simulink model "RAM_address_definition"  (R2020a)
settings: Solver=FixedStepDiscrete  StartTime=0.0  StopTime=840000  RelTol=1e-3
libraries: simulink x12, hdlsllib x8
settings Model: FPTRunName=FPA_Reference  PacingRate=40  Creator=BuccelliLab  LastModifiedBy=diflo
settings SolverCC: AutoInsertRateTranBlk=on  MinimalZcImpactIntegration=on
settings DataIOCC: LimitDataPoints=on  SaveOutput=off  SaveTime=off  ReturnWorkspaceOutputs=off
settings OptimizationCC: BlockReduction=off  ConditionallyExecuteInputs=off  DefaultParameterBehavior=Inlined  LifeSpan=inf
settings DebuggingCC: SignalRangeChecking=warning  ReadBeforeWriteMsg=DisableAll  WriteAfterWriteMsg=DisableAll  WriteAfterReadMsg=DisableAll  AlgebraicLoopMsg=error  MultiTaskDSMMsg=none  SingleTaskRateTransMsg=error  ParameterDowncastMsg=warning  ParameterOverflowMsg=warning  AllowSymbolicDim=off  StrictBusMsg=ErrorOnBusTreatedAsVector  SFUnexpectedBacktrackingDiag=warning  SFNoUnconditionalDefaultTransitionDiag=warning  SFExecutionAtInitializationDiag=none  ArithmeticOperatorsInVariantConditions=warning
settings HardwareCC: ProdBitPerPointer=32  ProdBitPerSizeT=32  ProdBitPerPtrDiffT=32  ProdLargestAtomicFloat=None  ProdIntDivRoundTo=Undefined  ProdEndianess=Unspecified  ProdWordSize=32  ProdHWDeviceType=ASIC/FPGA->ASIC/FPGA  TargetBitPerPointer=64  TargetBitPerSizeT=64  TargetBitPerPtrDiffT=64  TargetLongLongMode=on  TargetIntDivRoundTo=Zero  TargetEndianess=LittleEndian  TargetWordSize=64  TargetHWDeviceType=Custom Processor->MATLAB Host Computer  ProdEqTarget=off
settings ModelReferenceCC: UpdateModelReferenceTargets=IfOutOfDate
settings SFSimCC: SFSimEcho=off  SimUseLocalCustomCode=off  CustomCodeUndefinedFunction=UseInterfaceOnly
settings RTWCC: RTWUseLocalCustomCode=off
settings CodeAppCC: StateflowObjectComments=on
settings GRTTargetCC: TargetLangStandard=C89/C90 (ANSI)
settings ConfigComp: CovScope=ReferencedModels  CovMetricSettings=dw  CovHtmlReporting=on  CovSaveCumulativeToWorkspaceVar=on  CovSaveSingleToWorkspaceVar=on  CovExternalEMLEnable=off  CovSFcnEnable=off

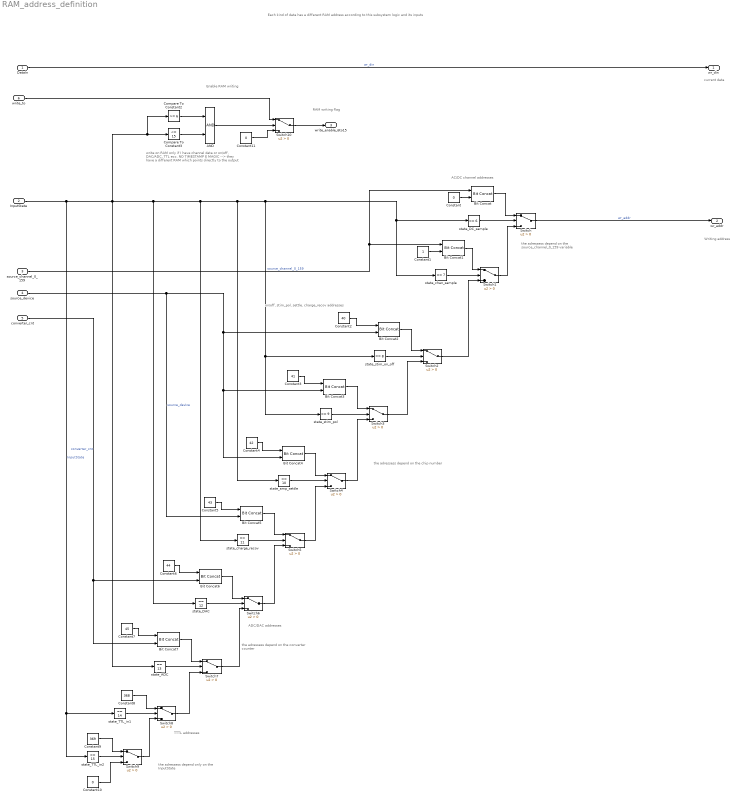
== system RAM_address_definition ==
  note: the adressess depend on the chip number
  note: Each kind of data has a different RAM
      | address according to this subsystem logic
      | and its inputs
  note: AC/DC channel addresses
  note: Writing address
  note: current data
  note: RAM writing flag
  note: write on RAM only if I have channel data or on/off,
      | DAC/ADC, TTL ecc.
      | NO TIMESTAMP E MAGIC --> they have a different
      | RAM which points directly to the output
  note: on/off, stim_pol, settle, charge_recov addresses
  note: ADC/DAC addresses
  note: TTTL addresses
  note: the adressess depend on the converter
      | counter
  note: the adressess depend only on the
      | InputState
  note: the adressess depend on the
      | source_channel_0_159 variable
  note: Enable RAM writing
  DataIn : Inport  OutDataTypeStr=uint16  PortDimensions=1  SampleTime=[1,0]
  InputState : Inport  Port=2  OutDataTypeStr=uint8  PortDimensions=1  SampleTime=[1,0]
  source_channel_0_159 : Inport  Port=3  OutDataTypeStr=uint8  PortDimensions=1  SampleTime=[1,0]
  source_device : Inport  Port=4  OutDataTypeStr=fixdt(0,3,0)  PortDimensions=1  SampleTime=[1,0]
  converter_cnt : Inport  Port=5  OutDataTypeStr=fixdt(0,3,0)  PortDimensions=1  SampleTime=[1,0]
  write_to : Inport  Port=6  OutDataTypeStr=boolean  PortDimensions=1  SampleTime=[1,0]
  AND : Logic  IconShape=distinctive  AllPortsSameDT=off  OutDataTypeStr=boolean
  Bit Concat{,1..7} (8 alike) : hdlsllib/Logic and Bit Operations/Bit Concat  numInputs=2
  Compare To Constant2 : simulink/Logic and Bit Operations/Compare To Constant  relop=>=  const=6  OutDataTypeStr=boolean
  Compare To Constant3 : simulink/Logic and Bit Operations/Compare To Constant  relop=<=  const=15  OutDataTypeStr=boolean
  Constant : Constant  Value=0  OutDataTypeStr=boolean  SampleTime=-1
  Constant1 : Constant  OutDataTypeStr=boolean  SampleTime=-1
  Constant10 : Constant  Value=0  OutDataTypeStr=fixdt(0,9)  SampleTime=-1
  Constant11 : Constant  Value=0  OutDataTypeStr=boolean  SampleTime=-1
  Constant2 : Constant  Value=40  OutDataTypeStr=fixdt(0,6)  SampleTime=-1
  Constant3 : Constant  Value=41  OutDataTypeStr=fixdt(0,6)  SampleTime=-1
  Constant4 : Constant  Value=42  OutDataTypeStr=fixdt(0,6)  SampleTime=-1
  Constant5 : Constant  Value=43  OutDataTypeStr=fixdt(0,6)  SampleTime=-1
  Constant6 : Constant  Value=44  OutDataTypeStr=fixdt(0,6)  SampleTime=-1
  Constant7 : Constant  Value=45  OutDataTypeStr=fixdt(0,6)  SampleTime=-1
  Constant8 : Constant  Value=368  OutDataTypeStr=fixdt(0,9)  SampleTime=-1
  Constant9 : Constant  Value=369  OutDataTypeStr=fixdt(0,9)  SampleTime=-1
  Switch{,1..10} (11 alike) : Switch  Criteria=u2 > Threshold
  state_ADC : simulink/Logic and Bit Operations/Compare To Constant  relop===  const=13  OutDataTypeStr=boolean
  state_DAC : simulink/Logic and Bit Operations/Compare To Constant  relop===  const=12  OutDataTypeStr=boolean
  state_DC_sample : simulink/Logic and Bit Operations/Compare To Constant  relop===  const=6  OutDataTypeStr=boolean
  state_TTL_in1 : simulink/Logic and Bit Operations/Compare To Constant  relop===  const=14  OutDataTypeStr=boolean
  state_TTL_in2 : simulink/Logic and Bit Operations/Compare To Constant  relop===  const=15  OutDataTypeStr=boolean
  state_amp_settle : simulink/Logic and Bit Operations/Compare To Constant  relop===  const=10  OutDataTypeStr=boolean
  state_chan_sample : simulink/Logic and Bit Operations/Compare To Constant  relop===  const=7  OutDataTypeStr=boolean
  state_charge_recov : simulink/Logic and Bit Operations/Compare To Constant  relop===  const=11  OutDataTypeStr=boolean
  state_stim_on_off : simulink/Logic and Bit Operations/Compare To Constant  relop===  const=8  OutDataTypeStr=boolean
  state_stim_pol : simulink/Logic and Bit Operations/Compare To Constant  relop===  const=9  OutDataTypeStr=boolean
  wr_din : Outport  OutDataTypeStr=uint16  PortDimensions=1  SampleTime=[1,0]  VectorParamsAs1DForOutWhenUnconnected=off
  wr_addr : Outport  Port=2  OutDataTypeStr=fixdt(0,9,0)  PortDimensions=1  SampleTime=[1,0]  VectorParamsAs1DForOutWhenUnconnected=off
  write_enable_6to15 : Outport  Port=3  OutDataTypeStr=boolean  PortDimensions=1  SampleTime=[1,0]  VectorParamsAs1DForOutWhenUnconnected=off
  wires:
  state_DC_sample/1 -> Switch/2
  source_channel_0_159/1 -> Bit Concat/1, Bit Concat1/1  "source_channel_0_159"
  Constant/1 -> Bit Concat/2
  Bit Concat/1 -> Switch/1
  state_chan_sample/1 -> Switch1/2
  Constant1/1 -> Bit Concat1/2
  Bit Concat1/1 -> Switch1/1
  Switch1/1 -> Switch/3
  Switch/1 -> wr_addr/1  "wr_addr"
  Constant2/1 -> Bit Concat2/1
  Bit Concat2/1 -> Switch2/1
  state_stim_on_off/1 -> Switch2/2
  Switch2/1 -> Switch1/3
  Constant3/1 -> Bit Concat3/1
  state_stim_pol/1 -> Switch3/2
  Bit Concat3/1 -> Switch3/1
  Switch3/1 -> Switch2/3
  Constant4/1 -> Bit Concat4/1
  state_amp_settle/1 -> Switch4/2
  Bit Concat4/1 -> Switch4/1
  Switch4/1 -> Switch3/3
  Bit Concat5/1 -> Switch5/1
  state_charge_recov/1 -> Switch5/2
  Constant5/1 -> Bit Concat5/1
  source_device/1 -> Bit Concat2/2, Bit Concat3/2, Bit Concat4/2, Bit Concat5/2  "source_device"
  Switch5/1 -> Switch4/3
  Bit Concat6/1 -> Switch6/1
  state_DAC/1 -> Switch6/2
  Constant6/1 -> Bit Concat6/1
  Switch6/1 -> Switch5/3
  converter_cnt/1 -> Bit Concat6/2, Bit Concat7/2  "converter_cnt"
  Bit Concat7/1 -> Switch7/1
  state_ADC/1 -> Switch7/2
  Constant7/1 -> Bit Concat7/1
  Switch7/1 -> Switch6/3
  state_TTL_in1/1 -> Switch8/2
  Constant8/1 -> Switch8/1
  Switch8/1 -> Switch7/3
  state_TTL_in2/1 -> Switch9/2
  Constant9/1 -> Switch9/1
  Switch9/1 -> Switch8/3
  Constant10/1 -> Switch9/3
  DataIn/1 -> wr_din/1  "wr_din"
  Compare To Constant3/1 -> AND/2
  InputState/1 -> Compare To Constant3/1, Compare To Constant2/1, state_DC_sample/1, state_chan_sample/1, state_stim_on_off/1, state_stim_pol/1, state_amp_settle/1, state_charge_recov/1, state_DAC/1, state_ADC/1, state_TTL_in2/1, state_TTL_in1/1  "InputState"
  AND/1 -> Switch10/2
  Switch10/1 -> write_enable_6to15/1
  write_to/1 -> Switch10/1
  Compare To Constant2/1 -> AND/1
  Constant11/1 -> Switch10/3
